simulink model "gm_sampleModel1525_sub"  (R2023a)
settings: Solver=VariableStepAuto  StartTime=0.0  StopTime=10.0  RelTol=1e-3
libraries: hdlsllib x2, simulink x1
settings Model: Creator=user1  LastModifiedBy=user1
settings OptimizationCC: BlockReduction=off  ConditionallyExecuteInputs=off
settings DebuggingCC: InheritedTsInSrcMsg=none

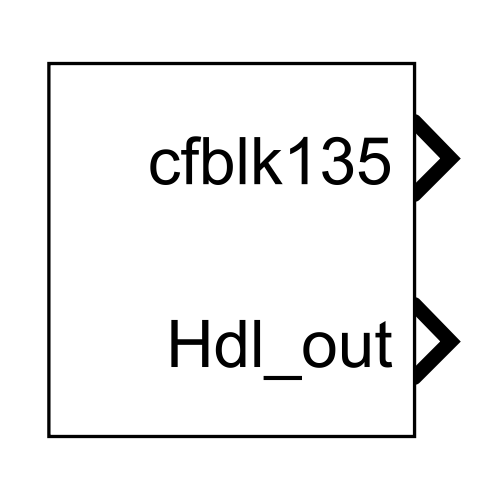
[thumbnail: Simulink's stored preview of the top-level diagram]
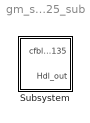
== system gm_sampleModel1525_sub ==
  Subsystem : Subsystem

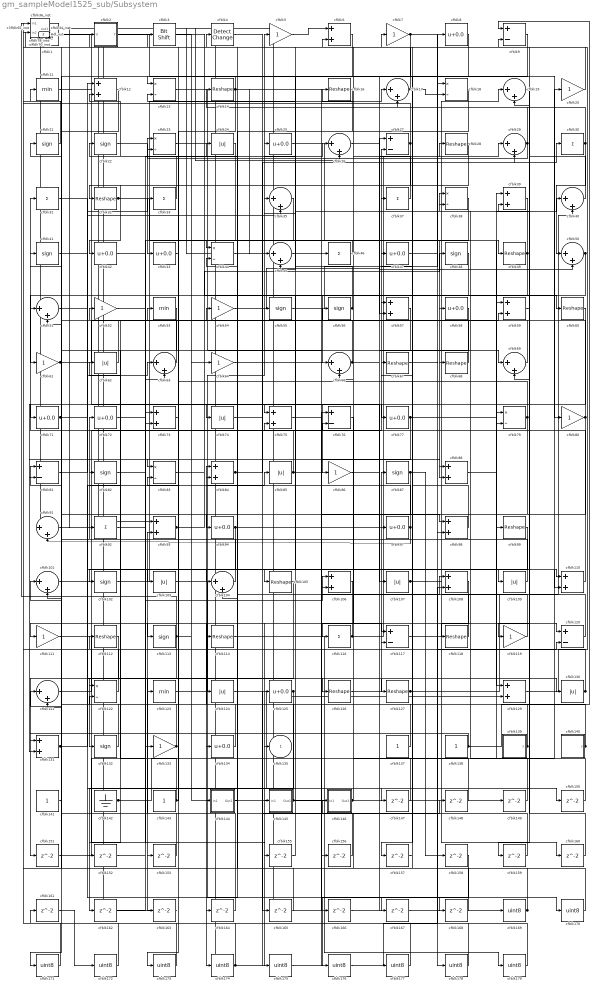
== system gm_sampleModel1525_sub/Subsystem ==
  cfblk1 : hdlsllib/Logic and Bit Operations/Bit Slice  lidx=7  ridx=0
  cfblk{17,19,26,29,35,40,45,50..51,63,66,69,91,101,104,121} (16 alike) : Sum  Inputs=|++  OutDataTypeStr=uint8
  cfblk{21..22,41,48,55..56,82,87,102,113,132} (11 alike) : Signum
  cfblk{24,62,74,85,103,107,109,124,130} (9 alike) : Abs  OutDataTypeStr=uint8  SaturateOnIntegerOverflow=off
  cfblk{14,16,28,32,49,60,67..68,99,105,112,114,118,126..127} (15 alike) : Reshape
  cfblk{6,12,39,57,59,73,75,84,88,93,98,106,108,110,129,131} (16 alike) : Sum  OutDataTypeStr=uint8
  cfblk10_inst : Subsystem
  cfblk11 : MinMax  OutDataTypeStr=uint8
  cfblk{5,7,20,52,54,61,64,80,86,111,119,133} (12 alike) : Gain  OutDataTypeStr=uint8
  cfblk115_inst : Subsystem
  cfblk{30..31,33,37,46,92,116} (7 alike) : Sum  Inputs=+  OutDataTypeStr=uint8
  cfblk{9,27,76,81,117,120} (6 alike) : Sum  Inputs=+-  OutDataTypeStr=uint8
  cfblk{13,18,23,38,44,79,83,122} (8 alike) : Product  Inputs=*/  OutDataTypeStr=uint8  RndMeth=Zero  SaturateOnIntegerOverflow=on
  cfblk123 : MinMax  OutDataTypeStr=uint8
  cfblk{8,25,42..43,47,58,71..72,77,94,97,125,134} (13 alike) : Bias  Bias=0.0  SaturateOnIntegerOverflow=off
  cfblk128_inst : Subsystem
  cfblk{137..138,141,143} (4 alike) : Constant  OutDataTypeStr=uint8  SampleTime=-1
  cfblk139 : Subsystem  mask(Counter Free-Running){NumBits=double(16), tsamp=double(-1)}
      mask prompts: NumBits "Simulink:masks:NumberOfBits_MP"; tsamp "Simulink:masks:SampleTime_MP"
      mask help: Simulink:masks:CounterFreeRunning_MD
  cfblk140 : Subsystem  mask(Counter Free-Running){NumBits=double(16), tsamp=double(-1)}
      mask prompts: NumBits "Simulink:masks:NumberOfBits_MP"; tsamp "Simulink:masks:SampleTime_MP"
      mask help: Simulink:masks:CounterFreeRunning_MD
  cfblk142 : Ground
  cfblk144 : Subsystem
  cfblk145 : Subsystem
  cfblk146 : Subsystem
  cfblk{147..153,155..168} (21 alike) : Delay  SampleTime=1
  cfblk15_inst : Subsystem
  cfblk{169..179} (11 alike) : DataTypeConversion  OutDataTypeStr=uint8  SaturateOnIntegerOverflow=off  RndMeth=Floor
  cfblk2 : Subsystem  mask(Detect Fall Negative){vinit=double(0), InputProcessing=Elements as channels (sample based), OutDataTypeStr=uint8}
      mask prompts: vinit "Simulink:masks:InitialCondition_MP"; InputProcessing "Simulink:masks:InputProcessing_MP"; OutDataTypeStr "Simulink:masks:OutputDataType_MP"
      mask help: Simulink:masks:DetectFallNegative_MD
      mask init:
      | InputProcessing = 'Elements as channels (sample based)';
      | OutDataTypeStr = 'uint8';
      | vinit = double(0);
      mask TypeOptions InputProcessing: Simulink:masks:ColumnsAsChannelsFrameBased | Simulink:masks:ElementsAsChannelsSampleBased
      mask TypeOptions OutDataTypeStr: Simulink:masks:uint8 | Simulink:masks:boolean
      mask Display: fprintf('U < 0\n&  NOT\nU/z < 0')
  cfblk3 : hdlsllib/Logic and Bit Operations/Bit Shift  mode=Shift Left Logical  N=0
  cfblk34_inst : Subsystem
  cfblk36_inst : Subsystem
  cfblk4 : simulink/Logic and Bit Operations/Detect Change  vinit=0  OutDataTypeStr=uint8
      settings: LibrarySourceBlock=|
      | hdlsllib/Logic and Bit
      | Operations/Detect
      | Change
  cfblk53 : MinMax  OutDataTypeStr=uint8
  cfblk65_inst : Subsystem
  cfblk70_inst : Subsystem
  cfblk78_inst : Subsystem
  cfblk135 : Outport  OutDataTypeStr=uint8  SampleTime=1  VectorParamsAs1DForOutWhenUnconnected=off
  Hdl_out : Outport  Port=2  OutDataTypeStr=uint8  SampleTime=1
  wires:
  cfblk1/1 -> cfblk75/1
  cfblk10_inst/1(out1) -> cfblk149/1
  cfblk101/1 -> cfblk109/1
  cfblk102/1 -> cfblk17/1
  cfblk103/1 -> cfblk168/1
  cfblk104/1 -> cfblk72/1
  cfblk105/1 -> cfblk163/1
  cfblk106/1 -> cfblk175/1
  cfblk107/1 -> cfblk19/2, cfblk19/1, cfblk160/1, cfblk158/1
  cfblk108/1 -> cfblk174/1
  cfblk109/1 -> cfblk78_inst/2(in2)
  cfblk11/1 -> cfblk86/1
  cfblk110/1 -> cfblk31/1
  cfblk111/1 -> cfblk153/1
  cfblk112/1 -> cfblk132/1
  cfblk113/1 -> cfblk10_inst/1(in1), cfblk64/1, cfblk151/1
  cfblk114/1 -> cfblk179/1
  cfblk115_inst/1(out1) -> cfblk93/1
  cfblk116/1 -> cfblk28/1, cfblk111/1
  cfblk117/1 -> cfblk120/1
  cfblk118/1 -> cfblk53/1
  cfblk119/1 -> cfblk22/1
  cfblk12/1 -> cfblk101/2
  cfblk120/1 -> cfblk39/2
  cfblk121/1 -> cfblk27/2
  cfblk122/1 -> cfblk101/1
  cfblk123/1 -> cfblk5/1
  cfblk124/1 -> cfblk147/1
  cfblk125/1 -> cfblk162/1, cfblk135/1
  cfblk126/1 -> cfblk87/1
  cfblk127/1 -> cfblk40/2, cfblk79/2
  cfblk128_inst/1(out1) -> cfblk129/2
  cfblk129/1 -> cfblk9/2
  cfblk13/1 -> cfblk156/1
  cfblk130/1 -> cfblk47/1, cfblk34_inst/2(in2)
  cfblk131/1 -> cfblk85/1, cfblk167/1
  cfblk132/1 -> cfblk21/1
  cfblk133/1 -> cfblk41/1, cfblk122/2
  cfblk134/1 -> cfblk23/1
  cfblk137/1 -> cfblk52/1
  cfblk138/1 -> cfblk9/1, cfblk131/1
  cfblk139/1(y) -> cfblk25/1, cfblk16/1, cfblk54/1
  cfblk14/1 -> cfblk98/1, cfblk45/1, cfblk83/1, cfblk13/1
  cfblk140/1(y) -> cfblk82/1, cfblk67/1
  cfblk141/1 -> cfblk51/2
  cfblk142/1 -> cfblk79/1, cfblk20/1
  cfblk143/1 -> cfblk112/1, cfblk83/2
  cfblk144/1(Out1) -> cfblk4/1
  cfblk145/1(Out1) -> cfblk84/1, cfblk128_inst/1(in1)
  cfblk146/1(Out1) -> cfblk76/2, Hdl_out/1
  cfblk147/1 -> cfblk6/2
  cfblk148/1 -> cfblk66/2
  cfblk149/1 -> cfblk39/1
  cfblk15_inst/1(out1) -> cfblk46/1
  cfblk150/1 -> cfblk38/1
  cfblk151/1 -> cfblk63/2
  cfblk152/1 -> cfblk73/1
  cfblk153/1 -> cfblk93/2
  cfblk155/1 -> cfblk75/2
  cfblk156/1 -> cfblk104/2
  cfblk157/1 -> cfblk57/1
  cfblk158/1 -> cfblk176/1
  cfblk159/1 -> cfblk35/1
  cfblk16/1 -> cfblk134/1
  cfblk160/1 -> cfblk69/2
  cfblk161/1 -> cfblk172/1
  cfblk162/1 -> cfblk106/1
  cfblk163/1 -> cfblk1/1
  cfblk164/1 -> cfblk81/1
  cfblk165/1 -> cfblk121/1
  cfblk166/1 -> cfblk50/2
  cfblk167/1 -> cfblk120/2
  cfblk168/1 -> cfblk117/2
  cfblk169/1 -> cfblk84/2, cfblk146/1(In1)
  cfblk17/1 -> cfblk34_inst/1(in1), cfblk18/2
  cfblk170/1 -> cfblk36_inst/1(in1)
  cfblk171/1 -> cfblk36_inst/2(in2)
  cfblk172/1 -> cfblk115_inst/2(in2)
  cfblk173/1 -> cfblk161/1
  cfblk174/1 -> cfblk125/1, cfblk115_inst/1(in1), cfblk148/1
  cfblk175/1 -> cfblk108/1
  cfblk176/1 -> cfblk108/2
  cfblk177/1 -> cfblk76/1
  cfblk178/1 -> cfblk65_inst/1(in1)
  cfblk179/1 -> cfblk65_inst/2(in2)
  cfblk18/1 -> cfblk164/1
  cfblk19/1 -> cfblk159/1
  cfblk2/1(Y) -> cfblk80/1
  cfblk20/1 -> cfblk78_inst/1(in1)
  cfblk21/1 -> cfblk70_inst/2(in2)
  cfblk22/1 -> cfblk43/1
  cfblk23/1 -> cfblk88/2
  cfblk24/1 -> cfblk73/2
  cfblk25/1 -> cfblk68/1
  cfblk26/1 -> cfblk49/1
  cfblk27/1 -> cfblk32/1, cfblk128_inst/2(in2)
  cfblk28/1 -> cfblk42/1
  cfblk29/1 -> cfblk14/1, cfblk23/2
  cfblk3/1 -> cfblk60/1
  cfblk30/1 -> cfblk50/1, cfblk17/2
  cfblk31/1 -> cfblk150/1
  cfblk32/1 -> cfblk99/1, cfblk166/1, cfblk165/1
  cfblk33/1 -> cfblk12/2
  cfblk34_inst/1(out1) -> cfblk91/1
  cfblk35/1 -> cfblk104/1
  cfblk36_inst/1(out1) -> cfblk169/1
  cfblk37/1 -> cfblk15_inst/2(in2)
  cfblk38/1 -> cfblk74/1
  cfblk39/1 -> cfblk38/2
  cfblk4/1 -> cfblk170/1
  cfblk40/1 -> cfblk70_inst/1(in1)
  cfblk41/1 -> cfblk126/1
  cfblk42/1 -> cfblk155/1
  cfblk43/1 -> cfblk113/1
  cfblk44/1 -> cfblk58/1
  cfblk45/1 -> cfblk88/1
  cfblk46/1 -> cfblk44/1
  cfblk47/1 -> cfblk8/1
  cfblk48/1 -> cfblk61/1
  cfblk49/1 -> cfblk121/2, cfblk105/1, cfblk10_inst/2(in2)
  cfblk5/1 -> cfblk6/1
  cfblk50/1 -> cfblk77/1, cfblk66/1
  cfblk51/1 -> cfblk35/2
  cfblk52/1 -> cfblk133/1
  cfblk53/1 -> cfblk122/1
  cfblk54/1 -> cfblk27/1
  cfblk55/1 -> cfblk18/1
  cfblk56/1 -> cfblk13/2, cfblk2/1(U)
  cfblk57/1 -> cfblk71/1
  cfblk58/1 -> cfblk152/1
  cfblk59/1 -> cfblk119/1
  cfblk6/1 -> cfblk51/1
  cfblk60/1 -> cfblk81/2
  cfblk61/1 -> cfblk97/1, cfblk56/1
  cfblk62/1 -> cfblk15_inst/1(in1)
  cfblk63/1 -> cfblk11/1
  cfblk64/1 -> cfblk110/1
  cfblk65_inst/1(out1) -> cfblk177/1
  cfblk66/1 -> cfblk69/1, cfblk55/1
  cfblk67/1 -> cfblk178/1
  cfblk68/1 -> cfblk12/1
  cfblk69/1 -> cfblk24/1
  cfblk7/1 -> cfblk45/2, cfblk110/2
  cfblk70_inst/1(out1) -> cfblk92/1
  cfblk71/1 -> cfblk124/1, cfblk106/2, cfblk33/1
  cfblk72/1 -> cfblk130/1
  cfblk73/1 -> cfblk123/1
  cfblk74/1 -> cfblk127/1
  cfblk75/1 -> cfblk117/1
  cfblk76/1 -> cfblk116/1
  cfblk77/1 -> cfblk40/1, cfblk131/2
  cfblk78_inst/1(out1) -> cfblk26/2
  cfblk79/1 -> cfblk3/1, cfblk103/1
  cfblk8/1 -> cfblk57/2
  cfblk80/1 -> cfblk94/1, cfblk7/1
  cfblk81/1 -> cfblk63/1
  cfblk82/1 -> cfblk26/1
  cfblk83/1 -> cfblk59/2
  cfblk84/1 -> cfblk29/2, cfblk114/1
  cfblk85/1 -> cfblk98/2, cfblk62/1
  cfblk86/1 -> cfblk30/1
  cfblk87/1 -> cfblk171/1, cfblk118/1
  cfblk88/1 -> cfblk129/1
  cfblk9/1 -> cfblk157/1
  cfblk91/1 -> cfblk144/1(In1)
  cfblk92/1 -> cfblk145/1(In1)
  cfblk93/1 -> cfblk59/1, cfblk48/1
  cfblk94/1 -> cfblk29/1, cfblk173/1, cfblk107/1
  cfblk97/1 -> cfblk91/2, cfblk44/2
  cfblk98/1 -> cfblk37/1
  cfblk99/1 -> cfblk102/1

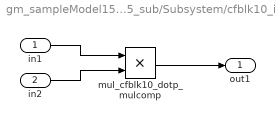
== system gm_sampleModel1525_sub/Subsystem/cfblk10_inst ==
  in1 : Inport  OutDataTypeStr=uint8  SampleTime=1
  in2 : Inport  Port=2  OutDataTypeStr=uint8  SampleTime=1
  mul_cfblk10_dotp_mulcomp : Product  Inputs=**  OutDataTypeStr=uint8  SampleTime=1
  out1 : Outport  OutDataTypeStr=uint8  SampleTime=1
  wires:
  in1/1 -> mul_cfblk10_dotp_mulcomp/1
  in2/1 -> mul_cfblk10_dotp_mulcomp/2
  mul_cfblk10_dotp_mulcomp/1 -> out1/1

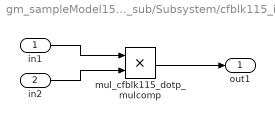
== system gm_sampleModel1525_sub/Subsystem/cfblk115_inst ==
  in1 : Inport  OutDataTypeStr=uint8  SampleTime=1
  in2 : Inport  Port=2  OutDataTypeStr=uint8  SampleTime=1
  mul_cfblk115_dotp_mulcomp : Product  Inputs=**  OutDataTypeStr=uint8  SampleTime=1
  out1 : Outport  OutDataTypeStr=uint8  SampleTime=1
  wires:
  in1/1 -> mul_cfblk115_dotp_mulcomp/1
  in2/1 -> mul_cfblk115_dotp_mulcomp/2
  mul_cfblk115_dotp_mulcomp/1 -> out1/1

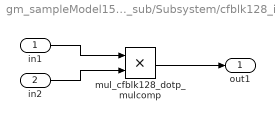
== system gm_sampleModel1525_sub/Subsystem/cfblk128_inst ==
  in1 : Inport  OutDataTypeStr=uint8  SampleTime=1
  in2 : Inport  Port=2  OutDataTypeStr=uint8  SampleTime=1
  mul_cfblk128_dotp_mulcomp : Product  Inputs=**  OutDataTypeStr=uint8  SampleTime=1
  out1 : Outport  OutDataTypeStr=uint8  SampleTime=1
  wires:
  in1/1 -> mul_cfblk128_dotp_mulcomp/1
  in2/1 -> mul_cfblk128_dotp_mulcomp/2
  mul_cfblk128_dotp_mulcomp/1 -> out1/1

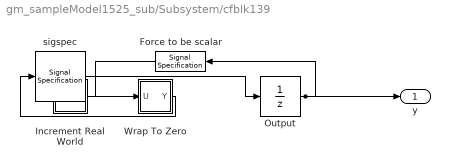
== system gm_sampleModel1525_sub/Subsystem/cfblk139 ==
  Force to be scalar : SignalSpecification  DisableCoverage=on  Dimensions=1
  Increment Real World : Subsystem  mask(Real World Value Increment){}
      mask help: Simulink:masks:RealWorldValueIncrement_MD
      mask Display: disp('V++')
  Output : UnitDelay  InitialCondition=0.0  SampleTime=tsamp  HasFrameUpgradeWarning=on
  Wrap To Zero : Subsystem  mask(Wrap To Zero){Threshold=double(65535)}
      mask prompts: Threshold "Simulink:masks:Threshold_MP"
      mask help: Simulink:masks:WrapToZero_MD
  sigspec : SignalSpecification  OutDataTypeStr=uint16  Dimensions=1
  y : Outport  SampleTime=1
  wires:
  Force to be scalar/1 -> Increment Real World/1(u)
  Increment Real World/1(y) -> Wrap To Zero/1(U)
  Output/1 -> Force to be scalar/1, y/1
  Wrap To Zero/1(Y) -> sigspec/1
  sigspec/1 -> Output/1

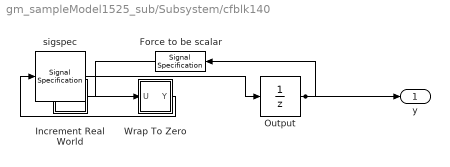
== system gm_sampleModel1525_sub/Subsystem/cfblk140 ==
  Force to be scalar : SignalSpecification  DisableCoverage=on  Dimensions=1
  Increment Real World : Subsystem  mask(Real World Value Increment){}
      mask help: Simulink:masks:RealWorldValueIncrement_MD
      mask Display: disp('V++')
  Output : UnitDelay  InitialCondition=0.0  SampleTime=tsamp  HasFrameUpgradeWarning=on
  Wrap To Zero : Subsystem  mask(Wrap To Zero){Threshold=double(65535)}
      mask prompts: Threshold "Simulink:masks:Threshold_MP"
      mask help: Simulink:masks:WrapToZero_MD
  sigspec : SignalSpecification  OutDataTypeStr=uint16  Dimensions=1
  y : Outport  SampleTime=1
  wires:
  Force to be scalar/1 -> Increment Real World/1(u)
  Increment Real World/1(y) -> Wrap To Zero/1(U)
  Output/1 -> Force to be scalar/1, y/1
  Wrap To Zero/1(Y) -> sigspec/1
  sigspec/1 -> Output/1

== system gm_sampleModel1525_sub/Subsystem/cfblk144 ==
  In1 : Inport  OutDataTypeStr=uint8  PortDimensions=1  SampleTime=1
  Out1 : Outport  SampleTime=1
  wires:
  In1/1 -> Out1/1

== system gm_sampleModel1525_sub/Subsystem/cfblk145 ==
  In1 : Inport  OutDataTypeStr=uint8  PortDimensions=1  SampleTime=1
  Out1 : Outport  SampleTime=1
  wires:
  In1/1 -> Out1/1

== system gm_sampleModel1525_sub/Subsystem/cfblk146 ==
  In1 : Inport  OutDataTypeStr=uint8  PortDimensions=1  SampleTime=1
  Out1 : Outport  SampleTime=1
  wires:
  In1/1 -> Out1/1

== system gm_sampleModel1525_sub/Subsystem/cfblk15_inst ==
  in1 : Inport  OutDataTypeStr=uint8  SampleTime=1
  in2 : Inport  Port=2  OutDataTypeStr=uint8  SampleTime=1
  mul_cfblk15_dotp_mulcomp : Product  Inputs=**  OutDataTypeStr=uint8  SampleTime=1
  out1 : Outport  OutDataTypeStr=uint8  SampleTime=1
  wires:
  in1/1 -> mul_cfblk15_dotp_mulcomp/1
  in2/1 -> mul_cfblk15_dotp_mulcomp/2
  mul_cfblk15_dotp_mulcomp/1 -> out1/1

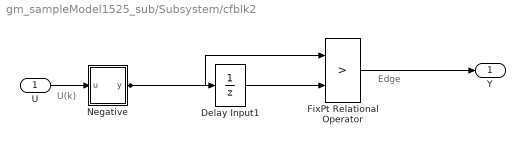
== system gm_sampleModel1525_sub/Subsystem/cfblk2 ==
  note: U(k)
  note: Edge
  U : Inport  OutDataTypeStr=uint8  SampleTime=1
  Delay Input1 : UnitDelay  Description=Store in Global RAM  DisableCoverage=on  InitialCondition=vinit  SampleTime=-1  HasFrameUpgradeWarning=on
  FixPt Relational Operator : RelationalOperator  Operator=>  OutDataTypeStr=fixdt(0, 8)  ZeroCross=off  InputSameDT=off
  Negative : Subsystem  mask(Compare To Zero){relop=<, OutDataTypeStr=boolean, ZeroCross=off}
      mask prompts: relop "Simulink:masks:Operator_MP"; OutDataTypeStr "Simulink:masks:OutputDataType_MP"; ZeroCross "Simulink:masks:EnableZerocrossingDetection_MP"
      mask help: Simulink:masks:CompareToZero_MD
      mask init:
      | OutDataTypeStr = 'boolean';
      | ZeroCross = 'off';
      | blkName = 'sampleModel1525_sub/Subsystem/cfblk2/Negative';
      | relop = '<';
      | setValue = 'boolean';
      mask TypeOptions relop: == | ~= | < | <= | >= | >
      mask TypeOptions OutDataTypeStr: Simulink:masks:uint8 | Simulink:masks:boolean
      mask Callback ZeroCross: sl('zeroCrossEnable', gcbh);
      mask Display: disp([relop,' 0'])
  Y : Outport  SampleTime=1
  wires:
  U/1 -> Negative/1(u)
  Delay Input1/1 -> FixPt Relational Operator/2
  FixPt Relational Operator/1 -> Y/1
  Negative/1(y) -> FixPt Relational Operator/1, Delay Input1/1

== system gm_sampleModel1525_sub/Subsystem/cfblk34_inst ==
  in1 : Inport  OutDataTypeStr=uint8  SampleTime=1
  in2 : Inport  Port=2  OutDataTypeStr=uint8  SampleTime=1
  mul_cfblk34_dotp_mulcomp : Product  Inputs=**  OutDataTypeStr=uint8  SampleTime=1
  out1 : Outport  OutDataTypeStr=uint8  SampleTime=1
  wires:
  in1/1 -> mul_cfblk34_dotp_mulcomp/1
  in2/1 -> mul_cfblk34_dotp_mulcomp/2
  mul_cfblk34_dotp_mulcomp/1 -> out1/1

== system gm_sampleModel1525_sub/Subsystem/cfblk36_inst ==
  in1 : Inport  OutDataTypeStr=uint8  SampleTime=1
  in2 : Inport  Port=2  OutDataTypeStr=uint8  SampleTime=1
  mul_cfblk36_dotp_mulcomp : Product  Inputs=**  OutDataTypeStr=uint8  SampleTime=1
  out1 : Outport  OutDataTypeStr=uint8  SampleTime=1
  wires:
  in1/1 -> mul_cfblk36_dotp_mulcomp/1
  in2/1 -> mul_cfblk36_dotp_mulcomp/2
  mul_cfblk36_dotp_mulcomp/1 -> out1/1

== system gm_sampleModel1525_sub/Subsystem/cfblk65_inst ==
  in1 : Inport  OutDataTypeStr=uint8  SampleTime=1
  in2 : Inport  Port=2  OutDataTypeStr=uint8  SampleTime=1
  mul_cfblk65_dotp_mulcomp : Product  Inputs=**  OutDataTypeStr=uint8  SampleTime=1
  out1 : Outport  OutDataTypeStr=uint8  SampleTime=1
  wires:
  in1/1 -> mul_cfblk65_dotp_mulcomp/1
  in2/1 -> mul_cfblk65_dotp_mulcomp/2
  mul_cfblk65_dotp_mulcomp/1 -> out1/1

== system gm_sampleModel1525_sub/Subsystem/cfblk70_inst ==
  in1 : Inport  OutDataTypeStr=uint8  SampleTime=1
  in2 : Inport  Port=2  OutDataTypeStr=uint8  SampleTime=1
  mul_cfblk70_dotp_mulcomp : Product  Inputs=**  OutDataTypeStr=uint8  SampleTime=1
  out1 : Outport  OutDataTypeStr=uint8  SampleTime=1
  wires:
  in1/1 -> mul_cfblk70_dotp_mulcomp/1
  in2/1 -> mul_cfblk70_dotp_mulcomp/2
  mul_cfblk70_dotp_mulcomp/1 -> out1/1

== system gm_sampleModel1525_sub/Subsystem/cfblk78_inst ==
  in1 : Inport  OutDataTypeStr=uint8  SampleTime=1
  in2 : Inport  Port=2  OutDataTypeStr=uint8  SampleTime=1
  mul_cfblk78_dotp_mulcomp : Product  Inputs=**  OutDataTypeStr=uint8  SampleTime=1
  out1 : Outport  OutDataTypeStr=uint8  SampleTime=1
  wires:
  in1/1 -> mul_cfblk78_dotp_mulcomp/1
  in2/1 -> mul_cfblk78_dotp_mulcomp/2
  mul_cfblk78_dotp_mulcomp/1 -> out1/1

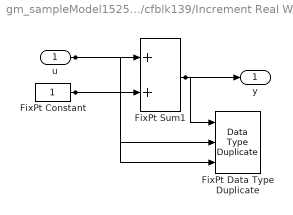
== system gm_sampleModel1525_sub/Subsystem/cfblk139/Increment Real World ==
  u : Inport  OutDataTypeStr=uint16  SampleTime=1
  FixPt Constant : Constant  DisableCoverage=on  OutDataTypeStr=Inherit: Inherit via back propagation  SampleTime=-1
  FixPt Data Type Duplicate : DataTypeDuplicate  DisableCoverage=on  NumInputPorts=3
  FixPt Sum1 : Sum  InputSameDT=on  OutDataTypeStr=Inherit: Inherit via back propagation  LockScale=on
  y : Outport  SampleTime=1
  wires:
  u/1 -> FixPt Sum1/1, FixPt Data Type Duplicate/2
  FixPt Constant/1 -> FixPt Sum1/2, FixPt Data Type Duplicate/3
  FixPt Sum1/1 -> FixPt Data Type Duplicate/1, y/1

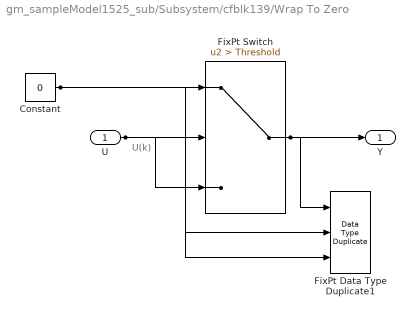
== system gm_sampleModel1525_sub/Subsystem/cfblk139/Wrap To Zero ==
  note: U(k)
  U : Inport  OutDataTypeStr=uint16  SampleTime=1
  Constant : Constant  DisableCoverage=on  Value=0  OutDataTypeStr=Inherit: Inherit via back propagation  SampleTime=-1
  FixPt Data Type Duplicate1 : DataTypeDuplicate  DisableCoverage=on  NumInputPorts=3
  FixPt Switch : Switch  Criteria=u2 > Threshold  Threshold=Threshold  OutDataTypeStr=Inherit: Inherit via back propagation  ZeroCross=off  SaturateOnIntegerOverflow=off  InputSameDT=off
  Y : Outport  SampleTime=1
  wires:
  U/1 -> FixPt Switch/3, FixPt Switch/2, FixPt Data Type Duplicate1/2
  Constant/1 -> FixPt Switch/1, FixPt Data Type Duplicate1/3
  FixPt Switch/1 -> FixPt Data Type Duplicate1/1, Y/1

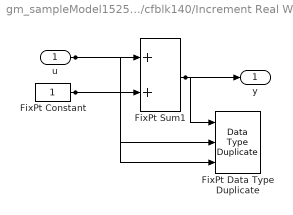
== system gm_sampleModel1525_sub/Subsystem/cfblk140/Increment Real World ==
  u : Inport  OutDataTypeStr=uint16  SampleTime=1
  FixPt Constant : Constant  DisableCoverage=on  OutDataTypeStr=Inherit: Inherit via back propagation  SampleTime=-1
  FixPt Data Type Duplicate : DataTypeDuplicate  DisableCoverage=on  NumInputPorts=3
  FixPt Sum1 : Sum  InputSameDT=on  OutDataTypeStr=Inherit: Inherit via back propagation  LockScale=on
  y : Outport  SampleTime=1
  wires:
  u/1 -> FixPt Sum1/1, FixPt Data Type Duplicate/2
  FixPt Constant/1 -> FixPt Sum1/2, FixPt Data Type Duplicate/3
  FixPt Sum1/1 -> FixPt Data Type Duplicate/1, y/1

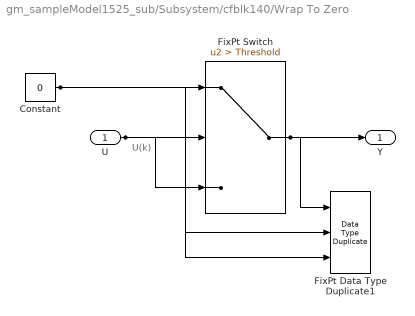
== system gm_sampleModel1525_sub/Subsystem/cfblk140/Wrap To Zero ==
  note: U(k)
  U : Inport  OutDataTypeStr=uint16  SampleTime=1
  Constant : Constant  DisableCoverage=on  Value=0  OutDataTypeStr=Inherit: Inherit via back propagation  SampleTime=-1
  FixPt Data Type Duplicate1 : DataTypeDuplicate  DisableCoverage=on  NumInputPorts=3
  FixPt Switch : Switch  Criteria=u2 > Threshold  Threshold=Threshold  OutDataTypeStr=Inherit: Inherit via back propagation  ZeroCross=off  SaturateOnIntegerOverflow=off  InputSameDT=off
  Y : Outport  SampleTime=1
  wires:
  U/1 -> FixPt Switch/3, FixPt Switch/2, FixPt Data Type Duplicate1/2
  Constant/1 -> FixPt Switch/1, FixPt Data Type Duplicate1/3
  FixPt Switch/1 -> FixPt Data Type Duplicate1/1, Y/1

== system gm_sampleModel1525_sub/Subsystem/cfblk2/Negative ==
  u : Inport  OutDataTypeStr=uint8  SampleTime=1
  Compare : RelationalOperator  Operator=<  OutDataTypeStr=boolean  ZeroCross=off
  Constant : Constant  DisableCoverage=on  Value=0  OutDataTypeStr=Inherit: Inherit via back propagation  SampleTime=-1  PreserveConstantTs=on
  y : Outport  SampleTime=1
  wires:
  u/1 -> Compare/1
  Compare/1 -> y/1
  Constant/1 -> Compare/2
